simulink model "orbit_propagator"  (R2023b)
settings: Solver=VariableStepAuto  StartTime=0.0  StopTime=10.0  RelTol=1e-3
model workspace: external: MAT-File orbitConstants.mat (data not in the file)
settings Model: Creator=annahylbert  LastModifiedBy=kristopherriordan

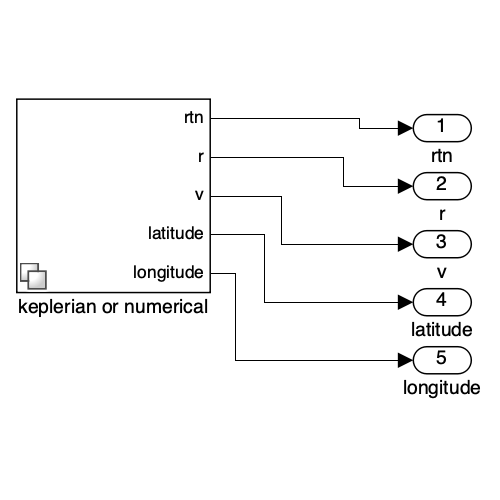
[thumbnail: Simulink's stored preview of the top-level diagram]
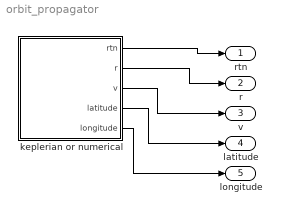
== system orbit_propagator ==
  keplerian or numerical : Subsystem  Variant=on
  rtn : Outport
  r : Outport  Port=2
  v : Outport  Port=3
  latitude : Outport  Port=4
  longitude : Outport  Port=5
  wires:
  keplerian or numerical/1(rtn) -> rtn/1
  keplerian or numerical/2(r) -> r/1
  keplerian or numerical/3(v) -> v/1
  keplerian or numerical/5(longitude) -> longitude/1
  keplerian or numerical/4(latitude) -> latitude/1

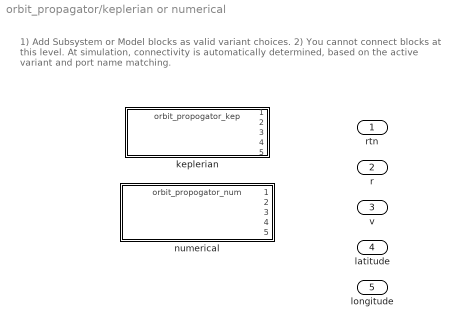
== system orbit_propagator/keplerian or numerical ==
  note: 1) Add Subsystem or Model blocks as valid variant choices.
      | 2) You cannot connect blocks at this level. At simulation, connectivity is automatically
      | determined, based on the active variant and port name matching.
  keplerian : ModelReference  ModelNameDialog=orbit_propogator_kep.slx  SimulationMode=Normal  VariantControl="orbitType==\"kep\""  ModelReferenceVersion=1.34
  numerical : ModelReference  ModelNameDialog=orbit_propogator_num.slx  SimulationMode=Normal  VariantControl="orbitType==\"num\""  ModelReferenceVersion=1.37
  rtn : Outport
  r : Outport  Port=2
  v : Outport  Port=3
  latitude : Outport  Port=4
  longitude : Outport  Port=5
